simulink model "SecRwRtStLgrstUpwdDnwdTrgtPosSelc"  (R2018b)
settings: Solver=FixedStepDiscrete  StartTime=0.0  StopTime=10.0  FixedStep=0.01  RelTol=1e-3
undefined symbols (not defined in the file or in its folder): KeSMSw4SAcsMd24SecRwRtStLegrstUpwdDnwdPos_Val, KeSMSw4SAcsMd24SecRwRtStLegrstUpwdDnwdPosMax_Val, KeSMSw4SAcsMd24SecRwRtStLegrstUpwdDnwdPosMin_Val, KeSMSw4SAcsMd26SecRwRtStLegrstUpwdDnwdPos_Val, KeSMSw4SAcsMd26SecRwRtStLegrstUpwdDnwdPosMax_Val, KeSMSw4SAcsMd26SecRwRtStLegrstUpwdDnwdPosMin_Val, KeSMSw4SLegrstCloseMdSecRwRtStLgrstUpwdDnwdPos_Val, KeSMSw4SLegrstCloseMdSecRwRtStLgrstUpwdDnwdPosMax_Val, KeSMSw4SLegrstCloseMdSecRwRtStLgrstUpwdDnwdPosMin_Val, KeSMSw4SLegrstOpenMdSecRwRtStLgrstUpwdDnwdPos_Val, KeSMSw4SLegrstOpenMdSecRwRtStLgrstUpwdDnwdPosMax_Val, KeSMSw4SLegrstOpenMdSecRwRtStLgrstUpwdDnwdPosMin_Val, KeSMSw4sLyingMDSecRwRtStLgrstUpwdPos_Val, KeSMSw4sLyingMDSecRwRtStLgrstUpwdPosMax_Val, KeSMSw4sLyingMDSecRwRtStLgrstUpwdPosMin_Val, KeSMSw4sRecoveryMDSecRwRtStLgrstUpwdPos_Val, KeSMSw4sRecoveryMDSecRwRtStLgrstUpwdPosMax_Val, KeSMSw4sRecoveryMDSecRwRtStLgrstUpwdPosMin_Val, KeSMSw4sVIPMDSecRwRtStLgrstUpwdPos_Val, KeSMSw4sVIPMDSecRwRtStLgrstUpwdPosMax_Val, KeSMSw4sVIPMDSecRwRtStLgrstUpwdPosMin_Val, KeSMSw6sAcsEntrySecRwRtStLgrstUpwdPos_Val, KeSMSw6sAcsEntrySecRwRtStLgrstUpwdPosMax_Val, KeSMSw6sAcsEntrySecRwRtStLgrstUpwdPosMin_Val, KeSMSw6sAcsExtSecRwRtStLgrstUpwdDnwdPos_Val, KeSMSw6sAcsExtSecRwRtStLgrstUpwdDnwdPosMax_Val, KeSMSw6sAcsExtSecRwRtStLgrstUpwdDnwdPosMin_Val, KeSMSw6sRecoveryMdSecRwRtStLgrstUpwdDnwdPos_Val, KeSMSw6sRecoveryMdSecRwRtStLgrstUpwdDnwdPosMax_Val, KeSMSw6sRecoveryMdSecRwRtStLgrstUpwdDnwdPosMin_Val, KeSMSw6sVIPSecRwRtStLgrstUpwdPos_Val, KeSMSw6sVIPSecRwRtStLgrstUpwdPosMax_Val, KeSMSw6sVIPSecRwRtStLgrstUpwdPosMin_Val, KeSMSwAcsEntrySecRwRtStLgrstUpwdPos_Val, KeSMSwAcsEntrySecRwRtStLgrstUpwdPosMax_Val, KeSMSwAcsEntrySecRwRtStLgrstUpwdPosMin_Val, KeSMSwAcsExtSecRwRtStLgrstUpwdDnwdPos_Val, KeSMSwAcsExtSecRwRtStLgrstUpwdDnwdPosMax_Val, KeSMSwAcsExtSecRwRtStLgrstUpwdDnwdPosMin_Val, KeSMSwAcsMd8SecRwRtStLgrstUpwdPos_Val, KeSMSwAcsMd8SecRwRtStLgrstUpwdPosMax_Val, KeSMSwAcsMd8SecRwRtStLgrstUpwdPosMin_Val, KeSMSwAcsMd9SecRwRtStLgrstUpwdPos_Val, KeSMSwAcsMd9SecRwRtStLgrstUpwdPosMax_Val, KeSMSwAcsMd9SecRwRtStLgrstUpwdPosMin_Val, KeSMSwRecoveryMdSecRwRtStLgrstUpwdDnwdPos_Val, KeSMSwRecoveryMdSecRwRtStLgrstUpwdDnwdPosMax_Val, KeSMSwRecoveryMdSecRwRtStLgrstUpwdDnwdPosMin_Val, KeSMSwVIPSecRwRtStLgrstUpwdPos_Val, KeSMSwVIPSecRwRtStLgrstUpwdPosMax_Val, KeSMSwVIPSecRwRtStLgrstUpwdPosMin_Val
libraries: TrgtPosSelcLib x12
settings Model: Creator=sn2xws  LastModifiedBy=sn2xws
settings Model: ModifiedHistory=|
  | 2023.8.1 V2.0.0 CR421790 增加模式21-26
  | 2024.7.8 V3.0.0 557模式流程V1.9
settings DataIOCC: SaveFormat=StructureWithTime
settings OptimizationCC: DefaultParameterBehavior=Inlined  EnhancedBackFolding=on  PassReuseOutputArgsAs=Individual arguments  ZeroExternalMemoryAtStartup=off  ZeroInternalMemoryAtStartup=off  OptimizeBlockOrder=speed  DifferentSizesBufferReuse=on  OptimizationCustomize=off
settings DebuggingCC: ParameterTunabilityLossMsg=error
settings ModelReferenceCC: ModelReferenceNumInstancesAllowed=Single
settings SFSimCC: MATLABDynamicMemAlloc=off
settings RTWCC: SystemTargetFile=autosar.tlc  GenCodeOnly=on  TemplateMakefile=ert_default_tmf  Description=AUTOSAR  GenerateReport=on  IncludeHyperlinkInReport=on  LaunchReport=on  GenerateTraceInfo=on  GenerateTraceReport=on  GenerateTraceReportSl=on  GenerateTraceReportSf=on  GenerateTraceReportEml=on
settings CodeAppCC: ForceParamTrailComments=on  IgnoreCustomStorageClasses=off  OperatorAnnotations=on  SimulinkDataObjDesc=on  SFDataObjDesc=on  InsertBlockDesc=on
settings STFCustomTargetCC: TargetLangStandard=C99 (ISO)  MultiwordLength=256  ParMdlRefBuildCompliant=on  CompOptLevelCompliant=on  IncludeMdlTerminateFcn=off  CombineOutputUpdateFcns=on  SuppressErrorStatus=on  ERTCustomFileBanners=on  SupportNonFinite=off  SupportComplex=off  SupportContinuousTime=off  SupportNonInlinedSFcns=off  RemoveResetFunc=on  MATLABClassNameForMDSCustomization=Simulink.SoftwareTarget.ERTCustomization  AutosarCompliant=on  UseToolchainInfoCompliant=on  LookupTableObjectStructAxisOrder=2,1,3,4,...  LUTObjectStructOrderEvenSpacing=Size,Table,Breakpoints  SystemTargetFile=autosar.tlc
settings ERTTargetCC: TargetLangStandard=C99 (ISO)  ConcurrentExecutionCompliant=off  IncludeMdlTerminateFcn=off  SuppressErrorStatus=on  SupportNonFinite=off  SupportComplex=off  ModelStepFunctionPrototypeControlCompliant=off  CPPClassGenCompliant=off  AutosarCompliant=on  LookupTableObjectStructAxisOrder=2,1,3,4,...  LUTObjectStructOrderEvenSpacing=Size,Table,Breakpoints  InlinedParameterPlacement=NonHierarchical  ERTCustomFileTemplate=example_file_process.tlc  ERTFilePackagingFormat=Compact

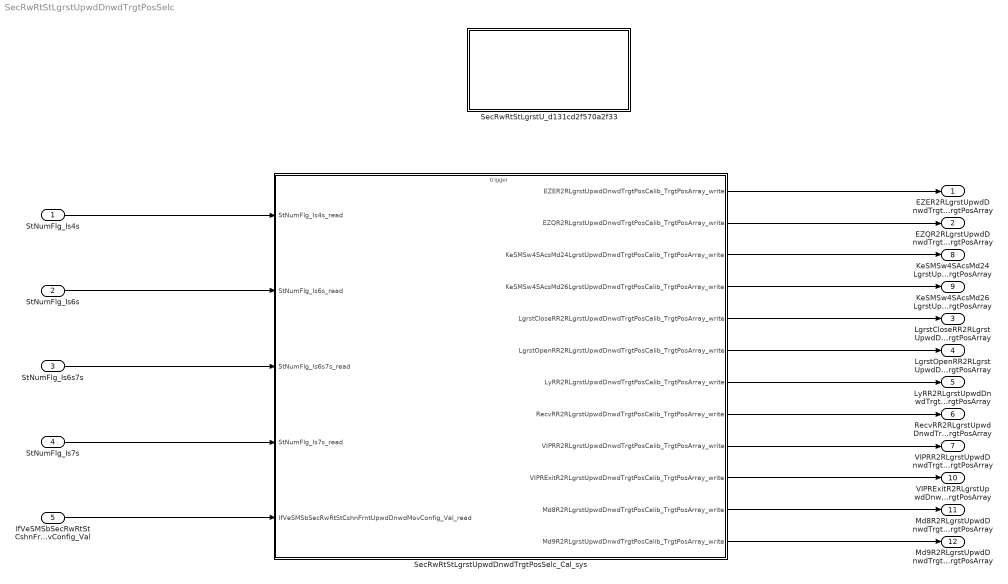
== system SecRwRtStLgrstUpwdDnwdTrgtPosSelc ==
  StNumFlg_Is4s : Inport  OutDataTypeStr=boolean  PortDimensions=1
  StNumFlg_Is6s : Inport  Port=2  OutDataTypeStr=boolean  PortDimensions=1
  StNumFlg_Is6s7s : Inport  Port=3  OutDataTypeStr=boolean  PortDimensions=1
  StNumFlg_Is7s : Inport  Port=4  OutDataTypeStr=boolean  PortDimensions=1
  IfVeSMSbSecRwRtStCshnFrntUpwdDnwdMovConfig_Val : Inport  Port=5  OutDataTypeStr=boolean  PortDimensions=1
  SecRwRtStLgrstU_d131cd2f570a2f33 : Subsystem
  SecRwRtStLgrstUpwdDnwdTrgtPosSelc_Cal_sys : Subsystem
  EZER2RLgrstUpwdDnwdTrgtPosCalib_TrgtPosArray : Outport  Description=|  OutDataTypeStr=uint16  PortDimensions=3
      | 0:Pos
      | 1:Max
      | 2:Min
  EZQR2RLgrstUpwdDnwdTrgtPosCalib_TrgtPosArray : Outport  Description=|  Port=2  OutDataTypeStr=uint16  PortDimensions=3
      | 0:Pos
      | 1:Max
      | 2:Min
  LgrstCloseRR2RLgrstUpwdDnwdTrgtPosCalib_TrgtPosArray : Outport  Description=|  Port=3  OutDataTypeStr=uint16  PortDimensions=3
      | 0:Pos
      | 1:Max
      | 2:Min
  LgrstOpenRR2RLgrstUpwdDnwdTrgtPosCalib_TrgtPosArray : Outport  Description=|  Port=4  OutDataTypeStr=uint16  PortDimensions=3
      | 0:Pos
      | 1:Max
      | 2:Min
  LyRR2RLgrstUpwdDnwdTrgtPosCalib_TrgtPosArray : Outport  Description=|  Port=5  OutDataTypeStr=uint16  PortDimensions=3
      | 0:Pos
      | 1:Max
      | 2:Min
  RecvRR2RLgrstUpwdDnwdTrgtPosCalib_TrgtPosArray : Outport  Description=|  Port=6  OutDataTypeStr=uint16  PortDimensions=3
      | 0:Pos
      | 1:Max
      | 2:Min
  VIPRR2RLgrstUpwdDnwdTrgtPosCalib_TrgtPosArray : Outport  Description=|  Port=7  OutDataTypeStr=uint16  PortDimensions=3
      | 0:Pos
      | 1:Max
      | 2:Min
  KeSMSw4SAcsMd24LgrstUpwdDnwdTrgtPosCalib_TrgtPosArray : Outport  Description=|  Port=8  OutDataTypeStr=uint16  PortDimensions=3
      | 0:Pos
      | 1:Max
      | 2:Min
  KeSMSw4SAcsMd26LgrstUpwdDnwdTrgtPosCalib_TrgtPosArray : Outport  Description=|  Port=9  OutDataTypeStr=uint16  PortDimensions=3
      | 0:Pos
      | 1:Max
      | 2:Min
  VIPRExitR2RLgrstUpwdDnwdTrgtPosCalib_TrgtPosArray : Outport  Description=|  Port=10  OutDataTypeStr=uint16  PortDimensions=3
      | 0:Pos
      | 1:Max
      | 2:Min
  Md8R2RLgrstUpwdDnwdTrgtPosCalib_TrgtPosArray : Outport  Description=|  Port=11  OutDataTypeStr=uint16  PortDimensions=3
      | 0:Pos
      | 1:Max
      | 2:Min
  Md9R2RLgrstUpwdDnwdTrgtPosCalib_TrgtPosArray : Outport  Description=|  Port=12  OutDataTypeStr=uint16  PortDimensions=3
      | 0:Pos
      | 1:Max
      | 2:Min
  wires:
  StNumFlg_Is4s/1 -> SecRwRtStLgrstUpwdDnwdTrgtPosSelc_Cal_sys/1(StNumFlg_Is4s_read)
  StNumFlg_Is6s/1 -> SecRwRtStLgrstUpwdDnwdTrgtPosSelc_Cal_sys/2(StNumFlg_Is6s_read)
  StNumFlg_Is6s7s/1 -> SecRwRtStLgrstUpwdDnwdTrgtPosSelc_Cal_sys/3(StNumFlg_Is6s7s_read)
  StNumFlg_Is7s/1 -> SecRwRtStLgrstUpwdDnwdTrgtPosSelc_Cal_sys/4(StNumFlg_Is7s_read)
  SecRwRtStLgrstUpwdDnwdTrgtPosSelc_Cal_sys/1(EZER2RLgrstUpwdDnwdTrgtPosCalib_TrgtPosArray_write) -> EZER2RLgrstUpwdDnwdTrgtPosCalib_TrgtPosArray/1
  SecRwRtStLgrstUpwdDnwdTrgtPosSelc_Cal_sys/2(EZQR2RLgrstUpwdDnwdTrgtPosCalib_TrgtPosArray_write) -> EZQR2RLgrstUpwdDnwdTrgtPosCalib_TrgtPosArray/1
  SecRwRtStLgrstUpwdDnwdTrgtPosSelc_Cal_sys/5(LgrstCloseRR2RLgrstUpwdDnwdTrgtPosCalib_TrgtPosArray_write) -> LgrstCloseRR2RLgrstUpwdDnwdTrgtPosCalib_TrgtPosArray/1
  SecRwRtStLgrstUpwdDnwdTrgtPosSelc_Cal_sys/6(LgrstOpenRR2RLgrstUpwdDnwdTrgtPosCalib_TrgtPosArray_write) -> LgrstOpenRR2RLgrstUpwdDnwdTrgtPosCalib_TrgtPosArray/1
  SecRwRtStLgrstUpwdDnwdTrgtPosSelc_Cal_sys/7(LyRR2RLgrstUpwdDnwdTrgtPosCalib_TrgtPosArray_write) -> LyRR2RLgrstUpwdDnwdTrgtPosCalib_TrgtPosArray/1
  SecRwRtStLgrstUpwdDnwdTrgtPosSelc_Cal_sys/8(RecvRR2RLgrstUpwdDnwdTrgtPosCalib_TrgtPosArray_write) -> RecvRR2RLgrstUpwdDnwdTrgtPosCalib_TrgtPosArray/1
  SecRwRtStLgrstUpwdDnwdTrgtPosSelc_Cal_sys/9(VIPRR2RLgrstUpwdDnwdTrgtPosCalib_TrgtPosArray_write) -> VIPRR2RLgrstUpwdDnwdTrgtPosCalib_TrgtPosArray/1
  SecRwRtStLgrstUpwdDnwdTrgtPosSelc_Cal_sys/3(KeSMSw4SAcsMd24LgrstUpwdDnwdTrgtPosCalib_TrgtPosArray_write) -> KeSMSw4SAcsMd24LgrstUpwdDnwdTrgtPosCalib_TrgtPosArray/1
  SecRwRtStLgrstUpwdDnwdTrgtPosSelc_Cal_sys/4(KeSMSw4SAcsMd26LgrstUpwdDnwdTrgtPosCalib_TrgtPosArray_write) -> KeSMSw4SAcsMd26LgrstUpwdDnwdTrgtPosCalib_TrgtPosArray/1
  IfVeSMSbSecRwRtStCshnFrntUpwdDnwdMovConfig_Val/1 -> SecRwRtStLgrstUpwdDnwdTrgtPosSelc_Cal_sys/5(IfVeSMSbSecRwRtStCshnFrntUpwdDnwdMovConfig_Val_read)
  SecRwRtStLgrstUpwdDnwdTrgtPosSelc_Cal_sys/10(VIPRExitR2RLgrstUpwdDnwdTrgtPosCalib_TrgtPosArray_write) -> VIPRExitR2RLgrstUpwdDnwdTrgtPosCalib_TrgtPosArray/1
  SecRwRtStLgrstUpwdDnwdTrgtPosSelc_Cal_sys/11(Md8R2RLgrstUpwdDnwdTrgtPosCalib_TrgtPosArray_write) -> Md8R2RLgrstUpwdDnwdTrgtPosCalib_TrgtPosArray/1
  SecRwRtStLgrstUpwdDnwdTrgtPosSelc_Cal_sys/12(Md9R2RLgrstUpwdDnwdTrgtPosCalib_TrgtPosArray_write) -> Md9R2RLgrstUpwdDnwdTrgtPosCalib_TrgtPosArray/1

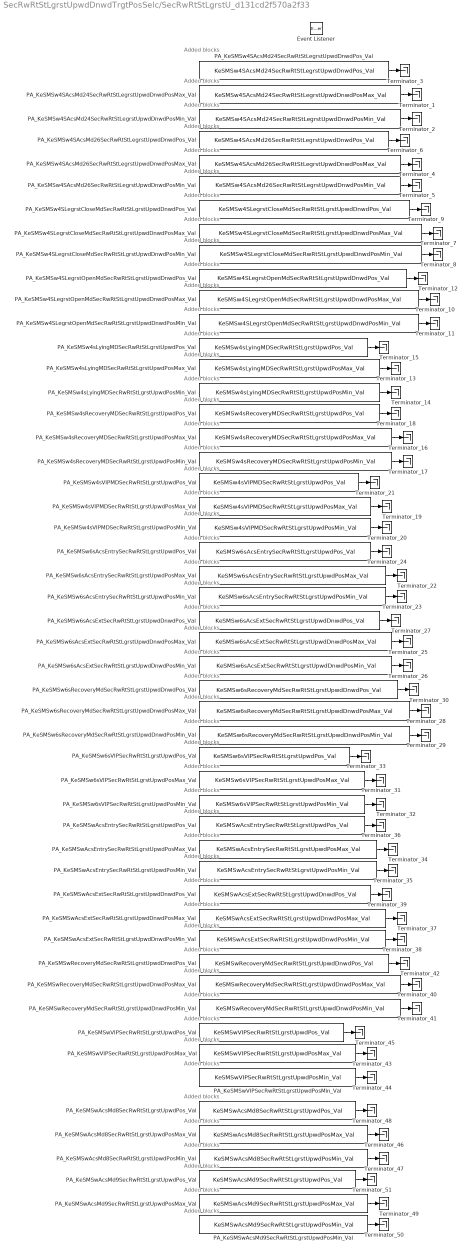
== system SecRwRtStLgrstUpwdDnwdTrgtPosSelc/SecRwRtStLgrstU_d131cd2f570a2f33 ==
  note: Added blocks
  note: Added blocks
  note: Added blocks
  note: Added blocks
  note: Added blocks
  note: Added blocks
  note: Added blocks
  note: Added blocks
  note: Added blocks
  note: Added blocks
  note: Added blocks
  note: Added blocks
  note: Added blocks
  note: Added blocks
  note: Added blocks
  note: Added blocks
  note: Added blocks
  note: Added blocks
  note: Added blocks
  note: Added blocks
  note: Added blocks
  note: Added blocks
  note: Added blocks
  note: Added blocks
  note: Added blocks
  note: Added blocks
  note: Added blocks
  note: Added blocks
  note: Added blocks
  note: Added blocks
  note: Added blocks
  note: Added blocks
  note: Added blocks
  note: Added blocks
  note: Added blocks
  note: Added blocks
  note: Added blocks
  note: Added blocks
  note: Added blocks
  note: Added blocks
  note: Added blocks
  note: Added blocks
  note: Added blocks
  note: Added blocks
  note: Added blocks
  note: Added blocks
  note: Added blocks
  note: Added blocks
  note: Added blocks
  note: Added blocks
  note: Added blocks
  Event Listener : EventListener  EventName=reset
  PA_KeSMSw4SAcsMd24SecRwRtStLegrstUpwdDnwdPosMax_Val : Constant  Value=KeSMSw4SAcsMd24SecRwRtStLegrstUpwdDnwdPosMax_Val
  PA_KeSMSw4SAcsMd24SecRwRtStLegrstUpwdDnwdPosMin_Val : Constant  Value=KeSMSw4SAcsMd24SecRwRtStLegrstUpwdDnwdPosMin_Val
  PA_KeSMSw4SAcsMd24SecRwRtStLegrstUpwdDnwdPos_Val : Constant  Value=KeSMSw4SAcsMd24SecRwRtStLegrstUpwdDnwdPos_Val
  PA_KeSMSw4SAcsMd26SecRwRtStLegrstUpwdDnwdPosMax_Val : Constant  Value=KeSMSw4SAcsMd26SecRwRtStLegrstUpwdDnwdPosMax_Val
  PA_KeSMSw4SAcsMd26SecRwRtStLegrstUpwdDnwdPosMin_Val : Constant  Value=KeSMSw4SAcsMd26SecRwRtStLegrstUpwdDnwdPosMin_Val
  PA_KeSMSw4SAcsMd26SecRwRtStLegrstUpwdDnwdPos_Val : Constant  Value=KeSMSw4SAcsMd26SecRwRtStLegrstUpwdDnwdPos_Val
  PA_KeSMSw4SLegrstCloseMdSecRwRtStLgrstUpwdDnwdPosMax_Val : Constant  Value=KeSMSw4SLegrstCloseMdSecRwRtStLgrstUpwdDnwdPosMax_Val
  PA_KeSMSw4SLegrstCloseMdSecRwRtStLgrstUpwdDnwdPosMin_Val : Constant  Value=KeSMSw4SLegrstCloseMdSecRwRtStLgrstUpwdDnwdPosMin_Val
  PA_KeSMSw4SLegrstCloseMdSecRwRtStLgrstUpwdDnwdPos_Val : Constant  Value=KeSMSw4SLegrstCloseMdSecRwRtStLgrstUpwdDnwdPos_Val
  PA_KeSMSw4SLegrstOpenMdSecRwRtStLgrstUpwdDnwdPosMax_Val : Constant  Value=KeSMSw4SLegrstOpenMdSecRwRtStLgrstUpwdDnwdPosMax_Val
  PA_KeSMSw4SLegrstOpenMdSecRwRtStLgrstUpwdDnwdPosMin_Val : Constant  Value=KeSMSw4SLegrstOpenMdSecRwRtStLgrstUpwdDnwdPosMin_Val
  PA_KeSMSw4SLegrstOpenMdSecRwRtStLgrstUpwdDnwdPos_Val : Constant  Value=KeSMSw4SLegrstOpenMdSecRwRtStLgrstUpwdDnwdPos_Val
  PA_KeSMSw4sLyingMDSecRwRtStLgrstUpwdPosMax_Val : Constant  Value=KeSMSw4sLyingMDSecRwRtStLgrstUpwdPosMax_Val
  PA_KeSMSw4sLyingMDSecRwRtStLgrstUpwdPosMin_Val : Constant  Value=KeSMSw4sLyingMDSecRwRtStLgrstUpwdPosMin_Val
  PA_KeSMSw4sLyingMDSecRwRtStLgrstUpwdPos_Val : Constant  Value=KeSMSw4sLyingMDSecRwRtStLgrstUpwdPos_Val
  PA_KeSMSw4sRecoveryMDSecRwRtStLgrstUpwdPosMax_Val : Constant  Value=KeSMSw4sRecoveryMDSecRwRtStLgrstUpwdPosMax_Val
  PA_KeSMSw4sRecoveryMDSecRwRtStLgrstUpwdPosMin_Val : Constant  Value=KeSMSw4sRecoveryMDSecRwRtStLgrstUpwdPosMin_Val
  PA_KeSMSw4sRecoveryMDSecRwRtStLgrstUpwdPos_Val : Constant  Value=KeSMSw4sRecoveryMDSecRwRtStLgrstUpwdPos_Val
  PA_KeSMSw4sVIPMDSecRwRtStLgrstUpwdPosMax_Val : Constant  Value=KeSMSw4sVIPMDSecRwRtStLgrstUpwdPosMax_Val
  PA_KeSMSw4sVIPMDSecRwRtStLgrstUpwdPosMin_Val : Constant  Value=KeSMSw4sVIPMDSecRwRtStLgrstUpwdPosMin_Val
  PA_KeSMSw4sVIPMDSecRwRtStLgrstUpwdPos_Val : Constant  Value=KeSMSw4sVIPMDSecRwRtStLgrstUpwdPos_Val
  PA_KeSMSw6sAcsEntrySecRwRtStLgrstUpwdPosMax_Val : Constant  Value=KeSMSw6sAcsEntrySecRwRtStLgrstUpwdPosMax_Val
  PA_KeSMSw6sAcsEntrySecRwRtStLgrstUpwdPosMin_Val : Constant  Value=KeSMSw6sAcsEntrySecRwRtStLgrstUpwdPosMin_Val
  PA_KeSMSw6sAcsEntrySecRwRtStLgrstUpwdPos_Val : Constant  Value=KeSMSw6sAcsEntrySecRwRtStLgrstUpwdPos_Val
  PA_KeSMSw6sAcsExtSecRwRtStLgrstUpwdDnwdPosMax_Val : Constant  Value=KeSMSw6sAcsExtSecRwRtStLgrstUpwdDnwdPosMax_Val
  PA_KeSMSw6sAcsExtSecRwRtStLgrstUpwdDnwdPosMin_Val : Constant  Value=KeSMSw6sAcsExtSecRwRtStLgrstUpwdDnwdPosMin_Val
  PA_KeSMSw6sAcsExtSecRwRtStLgrstUpwdDnwdPos_Val : Constant  Value=KeSMSw6sAcsExtSecRwRtStLgrstUpwdDnwdPos_Val
  PA_KeSMSw6sRecoveryMdSecRwRtStLgrstUpwdDnwdPosMax_Val : Constant  Value=KeSMSw6sRecoveryMdSecRwRtStLgrstUpwdDnwdPosMax_Val
  PA_KeSMSw6sRecoveryMdSecRwRtStLgrstUpwdDnwdPosMin_Val : Constant  Value=KeSMSw6sRecoveryMdSecRwRtStLgrstUpwdDnwdPosMin_Val
  PA_KeSMSw6sRecoveryMdSecRwRtStLgrstUpwdDnwdPos_Val : Constant  Value=KeSMSw6sRecoveryMdSecRwRtStLgrstUpwdDnwdPos_Val
  PA_KeSMSw6sVIPSecRwRtStLgrstUpwdPosMax_Val : Constant  Value=KeSMSw6sVIPSecRwRtStLgrstUpwdPosMax_Val
  PA_KeSMSw6sVIPSecRwRtStLgrstUpwdPosMin_Val : Constant  Value=KeSMSw6sVIPSecRwRtStLgrstUpwdPosMin_Val
  PA_KeSMSw6sVIPSecRwRtStLgrstUpwdPos_Val : Constant  Value=KeSMSw6sVIPSecRwRtStLgrstUpwdPos_Val
  PA_KeSMSwAcsEntrySecRwRtStLgrstUpwdPosMax_Val : Constant  Value=KeSMSwAcsEntrySecRwRtStLgrstUpwdPosMax_Val
  PA_KeSMSwAcsEntrySecRwRtStLgrstUpwdPosMin_Val : Constant  Value=KeSMSwAcsEntrySecRwRtStLgrstUpwdPosMin_Val
  PA_KeSMSwAcsEntrySecRwRtStLgrstUpwdPos_Val : Constant  Value=KeSMSwAcsEntrySecRwRtStLgrstUpwdPos_Val
  PA_KeSMSwAcsExtSecRwRtStLgrstUpwdDnwdPosMax_Val : Constant  Value=KeSMSwAcsExtSecRwRtStLgrstUpwdDnwdPosMax_Val
  PA_KeSMSwAcsExtSecRwRtStLgrstUpwdDnwdPosMin_Val : Constant  Value=KeSMSwAcsExtSecRwRtStLgrstUpwdDnwdPosMin_Val
  PA_KeSMSwAcsExtSecRwRtStLgrstUpwdDnwdPos_Val : Constant  Value=KeSMSwAcsExtSecRwRtStLgrstUpwdDnwdPos_Val
  PA_KeSMSwAcsMd8SecRwRtStLgrstUpwdPosMax_Val : Constant  Value=KeSMSwAcsMd8SecRwRtStLgrstUpwdPosMax_Val
  PA_KeSMSwAcsMd8SecRwRtStLgrstUpwdPosMin_Val : Constant  Value=KeSMSwAcsMd8SecRwRtStLgrstUpwdPosMin_Val
  PA_KeSMSwAcsMd8SecRwRtStLgrstUpwdPos_Val : Constant  Value=KeSMSwAcsMd8SecRwRtStLgrstUpwdPos_Val
  PA_KeSMSwAcsMd9SecRwRtStLgrstUpwdPosMax_Val : Constant  Value=KeSMSwAcsMd9SecRwRtStLgrstUpwdPosMax_Val
  PA_KeSMSwAcsMd9SecRwRtStLgrstUpwdPosMin_Val : Constant  Value=KeSMSwAcsMd9SecRwRtStLgrstUpwdPosMin_Val
  PA_KeSMSwAcsMd9SecRwRtStLgrstUpwdPos_Val : Constant  Value=KeSMSwAcsMd9SecRwRtStLgrstUpwdPos_Val
  PA_KeSMSwRecoveryMdSecRwRtStLgrstUpwdDnwdPosMax_Val : Constant  Value=KeSMSwRecoveryMdSecRwRtStLgrstUpwdDnwdPosMax_Val
  PA_KeSMSwRecoveryMdSecRwRtStLgrstUpwdDnwdPosMin_Val : Constant  Value=KeSMSwRecoveryMdSecRwRtStLgrstUpwdDnwdPosMin_Val
  PA_KeSMSwRecoveryMdSecRwRtStLgrstUpwdDnwdPos_Val : Constant  Value=KeSMSwRecoveryMdSecRwRtStLgrstUpwdDnwdPos_Val
  PA_KeSMSwVIPSecRwRtStLgrstUpwdPosMax_Val : Constant  Value=KeSMSwVIPSecRwRtStLgrstUpwdPosMax_Val
  PA_KeSMSwVIPSecRwRtStLgrstUpwdPosMin_Val : Constant  Value=KeSMSwVIPSecRwRtStLgrstUpwdPosMin_Val
  PA_KeSMSwVIPSecRwRtStLgrstUpwdPos_Val : Constant  Value=KeSMSwVIPSecRwRtStLgrstUpwdPos_Val
  Terminator_{1..51} (51 alike) : Terminator
  wires:
  PA_KeSMSw4SAcsMd24SecRwRtStLegrstUpwdDnwdPosMax_Val/1 -> Terminator_1/1
  PA_KeSMSw4SAcsMd24SecRwRtStLegrstUpwdDnwdPosMin_Val/1 -> Terminator_2/1
  PA_KeSMSw4SAcsMd24SecRwRtStLegrstUpwdDnwdPos_Val/1 -> Terminator_3/1
  PA_KeSMSw4SAcsMd26SecRwRtStLegrstUpwdDnwdPosMax_Val/1 -> Terminator_4/1
  PA_KeSMSw4SAcsMd26SecRwRtStLegrstUpwdDnwdPosMin_Val/1 -> Terminator_5/1
  PA_KeSMSw4SAcsMd26SecRwRtStLegrstUpwdDnwdPos_Val/1 -> Terminator_6/1
  PA_KeSMSw4SLegrstCloseMdSecRwRtStLgrstUpwdDnwdPosMax_Val/1 -> Terminator_7/1
  PA_KeSMSw4SLegrstCloseMdSecRwRtStLgrstUpwdDnwdPosMin_Val/1 -> Terminator_8/1
  PA_KeSMSw4SLegrstCloseMdSecRwRtStLgrstUpwdDnwdPos_Val/1 -> Terminator_9/1
  PA_KeSMSw4SLegrstOpenMdSecRwRtStLgrstUpwdDnwdPosMax_Val/1 -> Terminator_10/1
  PA_KeSMSw4SLegrstOpenMdSecRwRtStLgrstUpwdDnwdPosMin_Val/1 -> Terminator_11/1
  PA_KeSMSw4SLegrstOpenMdSecRwRtStLgrstUpwdDnwdPos_Val/1 -> Terminator_12/1
  PA_KeSMSw4sLyingMDSecRwRtStLgrstUpwdPosMax_Val/1 -> Terminator_13/1
  PA_KeSMSw4sLyingMDSecRwRtStLgrstUpwdPosMin_Val/1 -> Terminator_14/1
  PA_KeSMSw4sLyingMDSecRwRtStLgrstUpwdPos_Val/1 -> Terminator_15/1
  PA_KeSMSw4sRecoveryMDSecRwRtStLgrstUpwdPosMax_Val/1 -> Terminator_16/1
  PA_KeSMSw4sRecoveryMDSecRwRtStLgrstUpwdPosMin_Val/1 -> Terminator_17/1
  PA_KeSMSw4sRecoveryMDSecRwRtStLgrstUpwdPos_Val/1 -> Terminator_18/1
  PA_KeSMSw4sVIPMDSecRwRtStLgrstUpwdPosMax_Val/1 -> Terminator_19/1
  PA_KeSMSw4sVIPMDSecRwRtStLgrstUpwdPosMin_Val/1 -> Terminator_20/1
  PA_KeSMSw4sVIPMDSecRwRtStLgrstUpwdPos_Val/1 -> Terminator_21/1
  PA_KeSMSw6sAcsEntrySecRwRtStLgrstUpwdPosMax_Val/1 -> Terminator_22/1
  PA_KeSMSw6sAcsEntrySecRwRtStLgrstUpwdPosMin_Val/1 -> Terminator_23/1
  PA_KeSMSw6sAcsEntrySecRwRtStLgrstUpwdPos_Val/1 -> Terminator_24/1
  PA_KeSMSw6sAcsExtSecRwRtStLgrstUpwdDnwdPosMax_Val/1 -> Terminator_25/1
  PA_KeSMSw6sAcsExtSecRwRtStLgrstUpwdDnwdPosMin_Val/1 -> Terminator_26/1
  PA_KeSMSw6sAcsExtSecRwRtStLgrstUpwdDnwdPos_Val/1 -> Terminator_27/1
  PA_KeSMSw6sRecoveryMdSecRwRtStLgrstUpwdDnwdPosMax_Val/1 -> Terminator_28/1
  PA_KeSMSw6sRecoveryMdSecRwRtStLgrstUpwdDnwdPosMin_Val/1 -> Terminator_29/1
  PA_KeSMSw6sRecoveryMdSecRwRtStLgrstUpwdDnwdPos_Val/1 -> Terminator_30/1
  PA_KeSMSw6sVIPSecRwRtStLgrstUpwdPosMax_Val/1 -> Terminator_31/1
  PA_KeSMSw6sVIPSecRwRtStLgrstUpwdPosMin_Val/1 -> Terminator_32/1
  PA_KeSMSw6sVIPSecRwRtStLgrstUpwdPos_Val/1 -> Terminator_33/1
  PA_KeSMSwAcsEntrySecRwRtStLgrstUpwdPosMax_Val/1 -> Terminator_34/1
  PA_KeSMSwAcsEntrySecRwRtStLgrstUpwdPosMin_Val/1 -> Terminator_35/1
  PA_KeSMSwAcsEntrySecRwRtStLgrstUpwdPos_Val/1 -> Terminator_36/1
  PA_KeSMSwAcsExtSecRwRtStLgrstUpwdDnwdPosMax_Val/1 -> Terminator_37/1
  PA_KeSMSwAcsExtSecRwRtStLgrstUpwdDnwdPosMin_Val/1 -> Terminator_38/1
  PA_KeSMSwAcsExtSecRwRtStLgrstUpwdDnwdPos_Val/1 -> Terminator_39/1
  PA_KeSMSwRecoveryMdSecRwRtStLgrstUpwdDnwdPosMax_Val/1 -> Terminator_40/1
  PA_KeSMSwRecoveryMdSecRwRtStLgrstUpwdDnwdPosMin_Val/1 -> Terminator_41/1
  PA_KeSMSwRecoveryMdSecRwRtStLgrstUpwdDnwdPos_Val/1 -> Terminator_42/1
  PA_KeSMSwVIPSecRwRtStLgrstUpwdPosMax_Val/1 -> Terminator_43/1
  PA_KeSMSwVIPSecRwRtStLgrstUpwdPosMin_Val/1 -> Terminator_44/1
  PA_KeSMSwVIPSecRwRtStLgrstUpwdPos_Val/1 -> Terminator_45/1
  PA_KeSMSwAcsMd8SecRwRtStLgrstUpwdPosMax_Val/1 -> Terminator_46/1
  PA_KeSMSwAcsMd8SecRwRtStLgrstUpwdPosMin_Val/1 -> Terminator_47/1
  PA_KeSMSwAcsMd8SecRwRtStLgrstUpwdPos_Val/1 -> Terminator_48/1
  PA_KeSMSwAcsMd9SecRwRtStLgrstUpwdPosMax_Val/1 -> Terminator_49/1
  PA_KeSMSwAcsMd9SecRwRtStLgrstUpwdPosMin_Val/1 -> Terminator_50/1
  PA_KeSMSwAcsMd9SecRwRtStLgrstUpwdPos_Val/1 -> Terminator_51/1

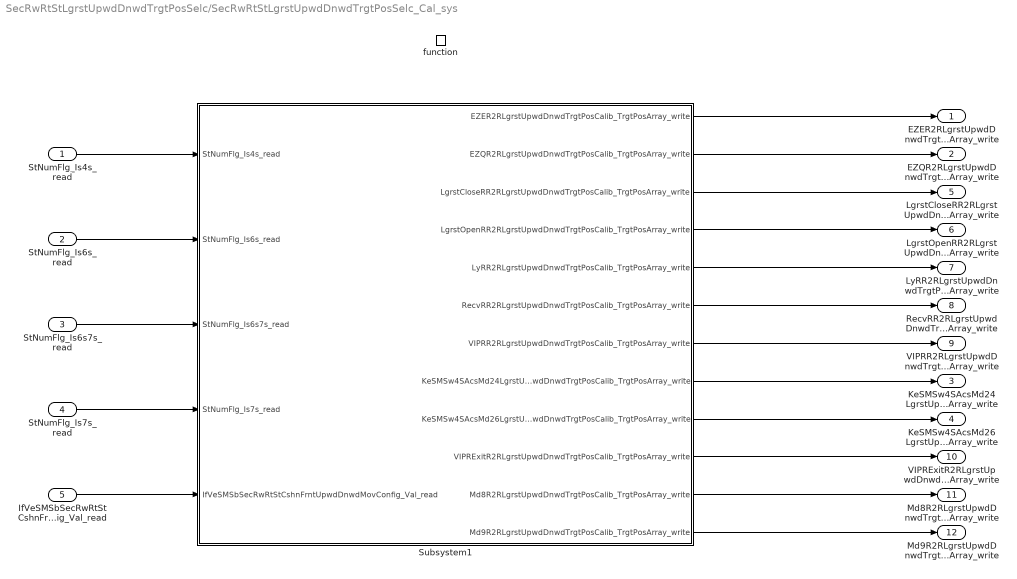
== system SecRwRtStLgrstUpwdDnwdTrgtPosSelc/SecRwRtStLgrstUpwdDnwdTrgtPosSelc_Cal_sys ==
  StNumFlg_Is4s_read : Inport
  StNumFlg_Is6s_read : Inport  Port=2
  StNumFlg_Is6s7s_read : Inport  Port=3
  StNumFlg_Is7s_read : Inport  Port=4
  IfVeSMSbSecRwRtStCshnFrntUpwdDnwdMovConfig_Val_read : Inport  Port=5
  function : TriggerPort  TriggerType=function-call  IsSimulinkFunction=on  FunctionName=SecRwRtStLgrstUpwdDnwdTrgtPosSelc_Cal  VariantControl=(inherit)
  Subsystem1 : Subsystem
  EZER2RLgrstUpwdDnwdTrgtPosCalib_TrgtPosArray_write : Outport
      settings: EnsureOutportIsVirtual=on
  EZQR2RLgrstUpwdDnwdTrgtPosCalib_TrgtPosArray_write : Outport  Port=2
      settings: EnsureOutportIsVirtual=on
  KeSMSw4SAcsMd24LgrstUpwdDnwdTrgtPosCalib_TrgtPosArray_write : Outport  Port=3
      settings: EnsureOutportIsVirtual=on
  KeSMSw4SAcsMd26LgrstUpwdDnwdTrgtPosCalib_TrgtPosArray_write : Outport  Port=4
      settings: EnsureOutportIsVirtual=on
  LgrstCloseRR2RLgrstUpwdDnwdTrgtPosCalib_TrgtPosArray_write : Outport  Port=5
      settings: EnsureOutportIsVirtual=on
  LgrstOpenRR2RLgrstUpwdDnwdTrgtPosCalib_TrgtPosArray_write : Outport  Port=6
      settings: EnsureOutportIsVirtual=on
  LyRR2RLgrstUpwdDnwdTrgtPosCalib_TrgtPosArray_write : Outport  Port=7
      settings: EnsureOutportIsVirtual=on
  RecvRR2RLgrstUpwdDnwdTrgtPosCalib_TrgtPosArray_write : Outport  Port=8
      settings: EnsureOutportIsVirtual=on
  VIPRR2RLgrstUpwdDnwdTrgtPosCalib_TrgtPosArray_write : Outport  Port=9
      settings: EnsureOutportIsVirtual=on
  VIPRExitR2RLgrstUpwdDnwdTrgtPosCalib_TrgtPosArray_write : Outport  Port=10
      settings: EnsureOutportIsVirtual=on
  Md8R2RLgrstUpwdDnwdTrgtPosCalib_TrgtPosArray_write : Outport  Port=11
      settings: EnsureOutportIsVirtual=on
  Md9R2RLgrstUpwdDnwdTrgtPosCalib_TrgtPosArray_write : Outport  Port=12
      settings: EnsureOutportIsVirtual=on
  wires:
  Subsystem1/1(EZER2RLgrstUpwdDnwdTrgtPosCalib_TrgtPosArray_write) -> EZER2RLgrstUpwdDnwdTrgtPosCalib_TrgtPosArray_write/1
  Subsystem1/2(EZQR2RLgrstUpwdDnwdTrgtPosCalib_TrgtPosArray_write) -> EZQR2RLgrstUpwdDnwdTrgtPosCalib_TrgtPosArray_write/1
  Subsystem1/7(VIPRR2RLgrstUpwdDnwdTrgtPosCalib_TrgtPosArray_write) -> VIPRR2RLgrstUpwdDnwdTrgtPosCalib_TrgtPosArray_write/1
  Subsystem1/8(KeSMSw4SAcsMd24LgrstUpwdDnwdTrgtPosCalib_TrgtPosArray_write) -> KeSMSw4SAcsMd24LgrstUpwdDnwdTrgtPosCalib_TrgtPosArray_write/1
  Subsystem1/4(LgrstOpenRR2RLgrstUpwdDnwdTrgtPosCalib_TrgtPosArray_write) -> LgrstOpenRR2RLgrstUpwdDnwdTrgtPosCalib_TrgtPosArray_write/1
  Subsystem1/5(LyRR2RLgrstUpwdDnwdTrgtPosCalib_TrgtPosArray_write) -> LyRR2RLgrstUpwdDnwdTrgtPosCalib_TrgtPosArray_write/1
  Subsystem1/6(RecvRR2RLgrstUpwdDnwdTrgtPosCalib_TrgtPosArray_write) -> RecvRR2RLgrstUpwdDnwdTrgtPosCalib_TrgtPosArray_write/1
  Subsystem1/9(KeSMSw4SAcsMd26LgrstUpwdDnwdTrgtPosCalib_TrgtPosArray_write) -> KeSMSw4SAcsMd26LgrstUpwdDnwdTrgtPosCalib_TrgtPosArray_write/1
  Subsystem1/3(LgrstCloseRR2RLgrstUpwdDnwdTrgtPosCalib_TrgtPosArray_write) -> LgrstCloseRR2RLgrstUpwdDnwdTrgtPosCalib_TrgtPosArray_write/1
  StNumFlg_Is4s_read/1 -> Subsystem1/1(StNumFlg_Is4s_read)
  StNumFlg_Is6s_read/1 -> Subsystem1/2(StNumFlg_Is6s_read)
  StNumFlg_Is6s7s_read/1 -> Subsystem1/3(StNumFlg_Is6s7s_read)
  StNumFlg_Is7s_read/1 -> Subsystem1/4(StNumFlg_Is7s_read)
  Subsystem1/10(VIPRExitR2RLgrstUpwdDnwdTrgtPosCalib_TrgtPosArray_write) -> VIPRExitR2RLgrstUpwdDnwdTrgtPosCalib_TrgtPosArray_write/1
  IfVeSMSbSecRwRtStCshnFrntUpwdDnwdMovConfig_Val_read/1 -> Subsystem1/5(IfVeSMSbSecRwRtStCshnFrntUpwdDnwdMovConfig_Val_read)
  Subsystem1/11(Md8R2RLgrstUpwdDnwdTrgtPosCalib_TrgtPosArray_write) -> Md8R2RLgrstUpwdDnwdTrgtPosCalib_TrgtPosArray_write/1
  Subsystem1/12(Md9R2RLgrstUpwdDnwdTrgtPosCalib_TrgtPosArray_write) -> Md9R2RLgrstUpwdDnwdTrgtPosCalib_TrgtPosArray_write/1

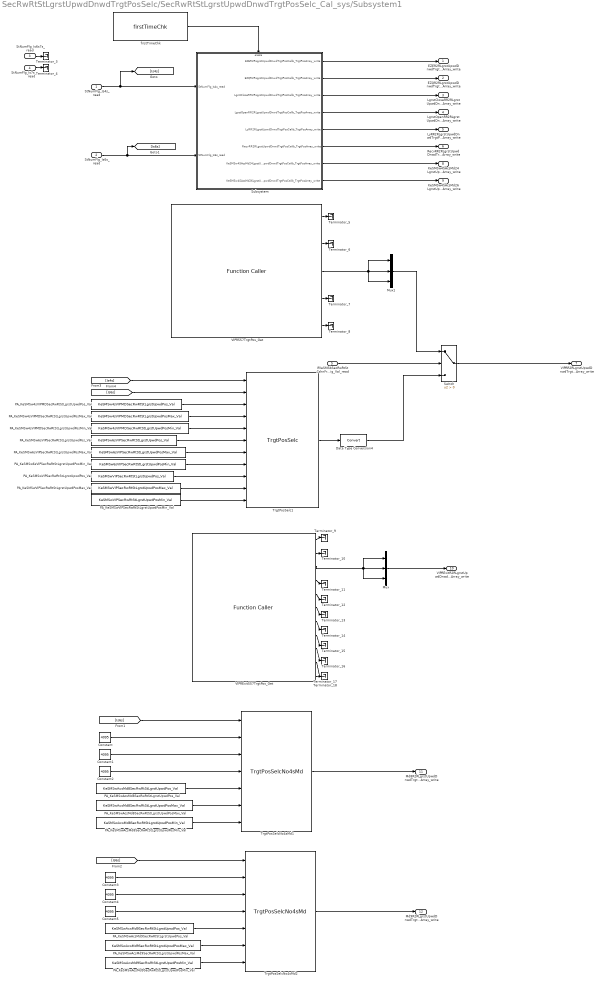
== system SecRwRtStLgrstUpwdDnwdTrgtPosSelc/SecRwRtStLgrstUpwdDnwdTrgtPosSelc_Cal_sys/Subsystem1 ==
  StNumFlg_Is4s_read : Inport
  StNumFlg_Is6s_read : Inport  Port=2
  StNumFlg_Is6s7s_read : Inport  Port=3
  StNumFlg_Is7s_read : Inport  Port=4
  IfVeSMSbSecRwRtStCshnFrntUpwdDnwdMovConfig_Val_read : Inport  Port=5
  Constant{,1..5} (6 alike) : Constant  Value=4095  OutDataTypeStr=uint16
  Data Type Conversion4 : DataTypeConversion
  Mux : Mux  Inputs=3
  Mux1 : Mux  Inputs=3
  PA_KeSMSw4sVIPMDSecRwRtStLgrstUpwdPosMax_Val : Constant  Value=KeSMSw4sVIPMDSecRwRtStLgrstUpwdPosMax_Val
  PA_KeSMSw4sVIPMDSecRwRtStLgrstUpwdPosMin_Val : Constant  Value=KeSMSw4sVIPMDSecRwRtStLgrstUpwdPosMin_Val
  PA_KeSMSw4sVIPMDSecRwRtStLgrstUpwdPos_Val : Constant  Value=KeSMSw4sVIPMDSecRwRtStLgrstUpwdPos_Val
  PA_KeSMSw6sVIPSecRwRtStLgrstUpwdPosMax_Val : Constant  Value=KeSMSw6sVIPSecRwRtStLgrstUpwdPosMax_Val
  PA_KeSMSw6sVIPSecRwRtStLgrstUpwdPosMin_Val : Constant  Value=KeSMSw6sVIPSecRwRtStLgrstUpwdPosMin_Val
  PA_KeSMSw6sVIPSecRwRtStLgrstUpwdPos_Val : Constant  Value=KeSMSw6sVIPSecRwRtStLgrstUpwdPos_Val
  PA_KeSMSwAcsMd8SecRwRtStLgrstUpwdPosMax_Val : Constant  Value=KeSMSwAcsMd8SecRwRtStLgrstUpwdPosMax_Val
  PA_KeSMSwAcsMd8SecRwRtStLgrstUpwdPosMin_Val : Constant  Value=KeSMSwAcsMd8SecRwRtStLgrstUpwdPosMin_Val
  PA_KeSMSwAcsMd8SecRwRtStLgrstUpwdPos_Val : Constant  Value=KeSMSwAcsMd8SecRwRtStLgrstUpwdPos_Val
  PA_KeSMSwAcsMd9SecRwRtStLgrstUpwdPosMax_Val : Constant  Value=KeSMSwAcsMd9SecRwRtStLgrstUpwdPosMax_Val
  PA_KeSMSwAcsMd9SecRwRtStLgrstUpwdPosMin_Val : Constant  Value=KeSMSwAcsMd9SecRwRtStLgrstUpwdPosMin_Val
  PA_KeSMSwAcsMd9SecRwRtStLgrstUpwdPos_Val : Constant  Value=KeSMSwAcsMd9SecRwRtStLgrstUpwdPos_Val
  PA_KeSMSwVIPSecRwRtStLgrstUpwdPosMax_Val : Constant  Value=KeSMSwVIPSecRwRtStLgrstUpwdPosMax_Val
  PA_KeSMSwVIPSecRwRtStLgrstUpwdPosMin_Val : Constant  Value=KeSMSwVIPSecRwRtStLgrstUpwdPosMin_Val
  PA_KeSMSwVIPSecRwRtStLgrstUpwdPos_Val : Constant  Value=KeSMSwVIPSecRwRtStLgrstUpwdPos_Val
  Subsystem : Subsystem
  Switch : Switch  Criteria=u2 > Threshold
  Terminator_{3..18} (16 alike) : Terminator
  TrgtPosSelc1 : TrgtPosSelcLib/TrgtPosSelc  SystemSampleTime=-1
  TrgtPosSelcNo4sMd1 : TrgtPosSelcLib/TrgtPosSelcNo4sMd  SystemSampleTime=-1
  TrgtPosSelcNo4sMd2 : TrgtPosSelcLib/TrgtPosSelcNo4sMd  SystemSampleTime=-1
  VIPR557TrgtPos_Get : FunctionCaller  FunctionPrototype=[SecRwLtStBkReclnTrgtPos,SecRwLtStZeroTrgtPos,SecRwLtStLgrstUpwdDnwdTrgtPos,SecRwLtStLgrstInwdOtwdTrgtPos,SecRwLtStFwdBkwdTrgtPos] = VIPR557TrgtPos_Get()  OutputArgumentSpecifications=uint16(1), uint16(1), uint16(1), uint16(1), uint16(1)
  VIPRExit557TrgtPos_Get : FunctionCaller  FunctionPrototype=[SecRwRtStBkReclnTrgtPos,SecRwRtStZeroTrgtPos,SecRwRtStLgrstUpwdDnwdTrgtPos,SecRwRtStLgrstInwdOtwdTrgtPos,ThdRwLtStBkReclnTrgtPos,ThdRwLtStFwdBkwdTrgtPos,ThdRwRtStBkReclnTrgtPos,ThdRwRtStFwdBkwdTrgtPos,PassStBkReclnTrgtPos,PassStFwdBkwdTrgtPos,SecRwRtStFwdBkwdTrgtPos] = VIPRExit557TrgtPos_Get()  OutputArgumentSpecifications=uint16(1), uint16(1), uint16(1), uint16(1), uint16(1), uint16(1), uint16(1), uint16(1), uint16(1), uint16(1), uint16(1)
  firstTimeChk : TrgtPosSelcLib/firstTimeChk  SystemSampleTime=-1
  EZER2RLgrstUpwdDnwdTrgtPosCalib_TrgtPosArray_write : Outport
      settings: EnsureOutportIsVirtual=on
  EZQR2RLgrstUpwdDnwdTrgtPosCalib_TrgtPosArray_write : Outport  Port=2
      settings: EnsureOutportIsVirtual=on
  LgrstCloseRR2RLgrstUpwdDnwdTrgtPosCalib_TrgtPosArray_write : Outport  Port=3
      settings: EnsureOutportIsVirtual=on
  LgrstOpenRR2RLgrstUpwdDnwdTrgtPosCalib_TrgtPosArray_write : Outport  Port=4
      settings: EnsureOutportIsVirtual=on
  LyRR2RLgrstUpwdDnwdTrgtPosCalib_TrgtPosArray_write : Outport  Port=5
      settings: EnsureOutportIsVirtual=on
  RecvRR2RLgrstUpwdDnwdTrgtPosCalib_TrgtPosArray_write : Outport  Port=6
      settings: EnsureOutportIsVirtual=on
  VIPRR2RLgrstUpwdDnwdTrgtPosCalib_TrgtPosArray_write : Outport  Port=7
      settings: EnsureOutportIsVirtual=on
  KeSMSw4SAcsMd24LgrstUpwdDnwdTrgtPosCalib_TrgtPosArray_write : Outport  Port=8
      settings: EnsureOutportIsVirtual=on
  KeSMSw4SAcsMd26LgrstUpwdDnwdTrgtPosCalib_TrgtPosArray_write : Outport  Port=9
      settings: EnsureOutportIsVirtual=on
  VIPRExitR2RLgrstUpwdDnwdTrgtPosCalib_TrgtPosArray_write : Outport  Port=10
      settings: EnsureOutportIsVirtual=on
  Md8R2RLgrstUpwdDnwdTrgtPosCalib_TrgtPosArray_write : Outport  Port=11
      settings: EnsureOutportIsVirtual=on
  Md9R2RLgrstUpwdDnwdTrgtPosCalib_TrgtPosArray_write : Outport  Port=12
      settings: EnsureOutportIsVirtual=on
  wires:
  StNumFlg_Is6s7s_read/1 -> Terminator_3/1
  Subsystem/2(EZQR2RLgrstUpwdDnwdTrgtPosCalib_TrgtPosArray_write) -> EZQR2RLgrstUpwdDnwdTrgtPosCalib_TrgtPosArray_write/1
  Subsystem/6(RecvRR2RLgrstUpwdDnwdTrgtPosCalib_TrgtPosArray_write) -> RecvRR2RLgrstUpwdDnwdTrgtPosCalib_TrgtPosArray_write/1
  Subsystem/3(LgrstCloseRR2RLgrstUpwdDnwdTrgtPosCalib_TrgtPosArray_write) -> LgrstCloseRR2RLgrstUpwdDnwdTrgtPosCalib_TrgtPosArray_write/1
  StNumFlg_Is7s_read/1 -> Terminator_4/1
  Subsystem/1(EZER2RLgrstUpwdDnwdTrgtPosCalib_TrgtPosArray_write) -> EZER2RLgrstUpwdDnwdTrgtPosCalib_TrgtPosArray_write/1
  Subsystem/5(LyRR2RLgrstUpwdDnwdTrgtPosCalib_TrgtPosArray_write) -> LyRR2RLgrstUpwdDnwdTrgtPosCalib_TrgtPosArray_write/1
  Subsystem/4(LgrstOpenRR2RLgrstUpwdDnwdTrgtPosCalib_TrgtPosArray_write) -> LgrstOpenRR2RLgrstUpwdDnwdTrgtPosCalib_TrgtPosArray_write/1
  firstTimeChk/1 -> Subsystem/Enable
  StNumFlg_Is6s_read/1 -> [Is6s], Subsystem/2(StNumFlg_Is6s_read)
  StNumFlg_Is4s_read/1 -> [Is4s], Subsystem/1(StNumFlg_Is4s_read)
  Subsystem/8(KeSMSw4SAcsMd26LgrstUpwdDnwdTrgtPosCalib_TrgtPosArray_write) -> KeSMSw4SAcsMd26LgrstUpwdDnwdTrgtPosCalib_TrgtPosArray_write/1
  Subsystem/7(KeSMSw4SAcsMd24LgrstUpwdDnwdTrgtPosCalib_TrgtPosArray_write) -> KeSMSw4SAcsMd24LgrstUpwdDnwdTrgtPosCalib_TrgtPosArray_write/1
  IfVeSMSbSecRwRtStCshnFrntUpwdDnwdMovConfig_Val_read/1 -> Switch/2
  Switch/1 -> VIPRR2RLgrstUpwdDnwdTrgtPosCalib_TrgtPosArray_write/1
  TrgtPosSelc1/1 -> Data Type Conversion4/1
  PA_KeSMSwVIPSecRwRtStLgrstUpwdPosMax_Val/1 -> TrgtPosSelc1/10
  PA_KeSMSw6sVIPSecRwRtStLgrstUpwdPosMin_Val/1 -> TrgtPosSelc1/8
  PA_KeSMSwVIPSecRwRtStLgrstUpwdPos_Val/1 -> TrgtPosSelc1/9
  PA_KeSMSw6sVIPSecRwRtStLgrstUpwdPosMax_Val/1 -> TrgtPosSelc1/7
  PA_KeSMSw6sVIPSecRwRtStLgrstUpwdPos_Val/1 -> TrgtPosSelc1/6
  [Is6s] -> TrgtPosSelc1/2
  PA_KeSMSw4sVIPMDSecRwRtStLgrstUpwdPosMax_Val/1 -> TrgtPosSelc1/4
  PA_KeSMSw4sVIPMDSecRwRtStLgrstUpwdPosMin_Val/1 -> TrgtPosSelc1/5
  PA_KeSMSw4sVIPMDSecRwRtStLgrstUpwdPos_Val/1 -> TrgtPosSelc1/3
  [Is4s] -> TrgtPosSelc1/1
  PA_KeSMSwVIPSecRwRtStLgrstUpwdPosMin_Val/1 -> TrgtPosSelc1/11
  Data Type Conversion4/1 -> Switch/3
  Mux/1 -> VIPRExitR2RLgrstUpwdDnwdTrgtPosCalib_TrgtPosArray_write/1
  VIPRExit557TrgtPos_Get/3 -> Mux/3, Mux/1, Mux/2
  Mux1/1 -> Switch/1
  VIPR557TrgtPos_Get/3 -> Mux1/3, Mux1/1, Mux1/2
  VIPR557TrgtPos_Get/1 -> Terminator_5/1
  VIPR557TrgtPos_Get/2 -> Terminator_6/1
  VIPR557TrgtPos_Get/4 -> Terminator_7/1
  VIPR557TrgtPos_Get/5 -> Terminator_8/1
  VIPRExit557TrgtPos_Get/1 -> Terminator_9/1
  VIPRExit557TrgtPos_Get/2 -> Terminator_10/1
  VIPRExit557TrgtPos_Get/4 -> Terminator_11/1
  VIPRExit557TrgtPos_Get/5 -> Terminator_12/1
  VIPRExit557TrgtPos_Get/6 -> Terminator_13/1
  VIPRExit557TrgtPos_Get/7 -> Terminator_14/1
  VIPRExit557TrgtPos_Get/8 -> Terminator_15/1
  VIPRExit557TrgtPos_Get/9 -> Terminator_16/1
  VIPRExit557TrgtPos_Get/10 -> Terminator_17/1
  VIPRExit557TrgtPos_Get/11 -> Terminator_18/1
  TrgtPosSelcNo4sMd1/1 -> Md8R2RLgrstUpwdDnwdTrgtPosCalib_TrgtPosArray_write/1
  TrgtPosSelcNo4sMd2/1 -> Md9R2RLgrstUpwdDnwdTrgtPosCalib_TrgtPosArray_write/1
  [Is6s] -> TrgtPosSelcNo4sMd1/1
  [Is6s] -> TrgtPosSelcNo4sMd2/1
  Constant/1 -> TrgtPosSelcNo4sMd1/2
  Constant1/1 -> TrgtPosSelcNo4sMd1/3
  Constant2/1 -> TrgtPosSelcNo4sMd1/4
  PA_KeSMSwAcsMd8SecRwRtStLgrstUpwdPos_Val/1 -> TrgtPosSelcNo4sMd1/5
  PA_KeSMSwAcsMd8SecRwRtStLgrstUpwdPosMax_Val/1 -> TrgtPosSelcNo4sMd1/6
  PA_KeSMSwAcsMd8SecRwRtStLgrstUpwdPosMin_Val/1 -> TrgtPosSelcNo4sMd1/7
  Constant5/1 -> TrgtPosSelcNo4sMd2/4
  Constant4/1 -> TrgtPosSelcNo4sMd2/3
  Constant3/1 -> TrgtPosSelcNo4sMd2/2
  PA_KeSMSwAcsMd9SecRwRtStLgrstUpwdPos_Val/1 -> TrgtPosSelcNo4sMd2/5
  PA_KeSMSwAcsMd9SecRwRtStLgrstUpwdPosMax_Val/1 -> TrgtPosSelcNo4sMd2/6
  PA_KeSMSwAcsMd9SecRwRtStLgrstUpwdPosMin_Val/1 -> TrgtPosSelcNo4sMd2/7

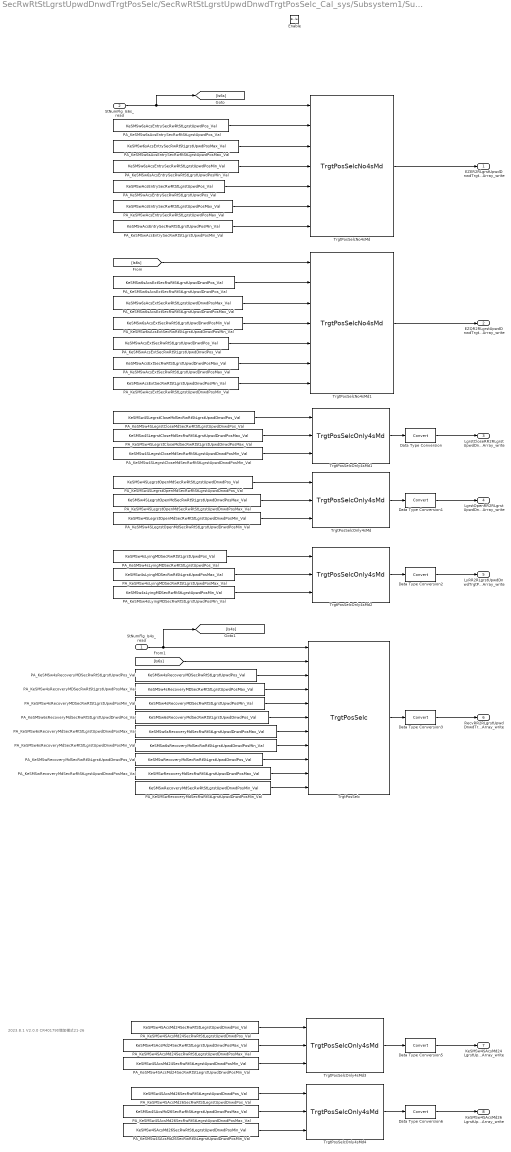
== system SecRwRtStLgrstUpwdDnwdTrgtPosSelc/SecRwRtStLgrstUpwdDnwdTrgtPosSelc_Cal_sys/Subsystem1/Subsystem ==
  note: 2023.8.1 V2.0.0 CR401790 增加模式21-26
  StNumFlg_Is4s_read : Inport
  StNumFlg_Is6s_read : Inport  Port=2
  Enable : EnablePort
  Data Type Conversion{,1..3,5..6} (6 alike) : DataTypeConversion
  PA_KeSMSw4SAcsMd24SecRwRtStLegrstUpwdDnwdPosMax_Val : Constant  Value=KeSMSw4SAcsMd24SecRwRtStLegrstUpwdDnwdPosMax_Val
  PA_KeSMSw4SAcsMd24SecRwRtStLegrstUpwdDnwdPosMin_Val : Constant  Value=KeSMSw4SAcsMd24SecRwRtStLegrstUpwdDnwdPosMin_Val
  PA_KeSMSw4SAcsMd24SecRwRtStLegrstUpwdDnwdPos_Val : Constant  Value=KeSMSw4SAcsMd24SecRwRtStLegrstUpwdDnwdPos_Val
  PA_KeSMSw4SAcsMd26SecRwRtStLegrstUpwdDnwdPosMax_Val : Constant  Value=KeSMSw4SAcsMd26SecRwRtStLegrstUpwdDnwdPosMax_Val
  PA_KeSMSw4SAcsMd26SecRwRtStLegrstUpwdDnwdPosMin_Val : Constant  Value=KeSMSw4SAcsMd26SecRwRtStLegrstUpwdDnwdPosMin_Val
  PA_KeSMSw4SAcsMd26SecRwRtStLegrstUpwdDnwdPos_Val : Constant  Value=KeSMSw4SAcsMd26SecRwRtStLegrstUpwdDnwdPos_Val
  PA_KeSMSw4SLegrstCloseMdSecRwRtStLgrstUpwdDnwdPosMax_Val : Constant  Value=KeSMSw4SLegrstCloseMdSecRwRtStLgrstUpwdDnwdPosMax_Val
  PA_KeSMSw4SLegrstCloseMdSecRwRtStLgrstUpwdDnwdPosMin_Val : Constant  Value=KeSMSw4SLegrstCloseMdSecRwRtStLgrstUpwdDnwdPosMin_Val
  PA_KeSMSw4SLegrstCloseMdSecRwRtStLgrstUpwdDnwdPos_Val : Constant  Value=KeSMSw4SLegrstCloseMdSecRwRtStLgrstUpwdDnwdPos_Val
  PA_KeSMSw4SLegrstOpenMdSecRwRtStLgrstUpwdDnwdPosMax_Val : Constant  Value=KeSMSw4SLegrstOpenMdSecRwRtStLgrstUpwdDnwdPosMax_Val
  PA_KeSMSw4SLegrstOpenMdSecRwRtStLgrstUpwdDnwdPosMin_Val : Constant  Value=KeSMSw4SLegrstOpenMdSecRwRtStLgrstUpwdDnwdPosMin_Val
  PA_KeSMSw4SLegrstOpenMdSecRwRtStLgrstUpwdDnwdPos_Val : Constant  Value=KeSMSw4SLegrstOpenMdSecRwRtStLgrstUpwdDnwdPos_Val
  PA_KeSMSw4sLyingMDSecRwRtStLgrstUpwdPosMax_Val : Constant  Value=KeSMSw4sLyingMDSecRwRtStLgrstUpwdPosMax_Val
  PA_KeSMSw4sLyingMDSecRwRtStLgrstUpwdPosMin_Val : Constant  Value=KeSMSw4sLyingMDSecRwRtStLgrstUpwdPosMin_Val
  PA_KeSMSw4sLyingMDSecRwRtStLgrstUpwdPos_Val : Constant  Value=KeSMSw4sLyingMDSecRwRtStLgrstUpwdPos_Val
  PA_KeSMSw4sRecoveryMDSecRwRtStLgrstUpwdPosMax_Val : Constant  Value=KeSMSw4sRecoveryMDSecRwRtStLgrstUpwdPosMax_Val
  PA_KeSMSw4sRecoveryMDSecRwRtStLgrstUpwdPosMin_Val : Constant  Value=KeSMSw4sRecoveryMDSecRwRtStLgrstUpwdPosMin_Val
  PA_KeSMSw4sRecoveryMDSecRwRtStLgrstUpwdPos_Val : Constant  Value=KeSMSw4sRecoveryMDSecRwRtStLgrstUpwdPos_Val
  PA_KeSMSw6sAcsEntrySecRwRtStLgrstUpwdPosMax_Val : Constant  Value=KeSMSw6sAcsEntrySecRwRtStLgrstUpwdPosMax_Val
  PA_KeSMSw6sAcsEntrySecRwRtStLgrstUpwdPosMin_Val : Constant  Value=KeSMSw6sAcsEntrySecRwRtStLgrstUpwdPosMin_Val
  PA_KeSMSw6sAcsEntrySecRwRtStLgrstUpwdPos_Val : Constant  Value=KeSMSw6sAcsEntrySecRwRtStLgrstUpwdPos_Val
  PA_KeSMSw6sAcsExtSecRwRtStLgrstUpwdDnwdPosMax_Val : Constant  Value=KeSMSw6sAcsExtSecRwRtStLgrstUpwdDnwdPosMax_Val
  PA_KeSMSw6sAcsExtSecRwRtStLgrstUpwdDnwdPosMin_Val : Constant  Value=KeSMSw6sAcsExtSecRwRtStLgrstUpwdDnwdPosMin_Val
  PA_KeSMSw6sAcsExtSecRwRtStLgrstUpwdDnwdPos_Val : Constant  Value=KeSMSw6sAcsExtSecRwRtStLgrstUpwdDnwdPos_Val
  PA_KeSMSw6sRecoveryMdSecRwRtStLgrstUpwdDnwdPosMax_Val : Constant  Value=KeSMSw6sRecoveryMdSecRwRtStLgrstUpwdDnwdPosMax_Val
  PA_KeSMSw6sRecoveryMdSecRwRtStLgrstUpwdDnwdPosMin_Val : Constant  Value=KeSMSw6sRecoveryMdSecRwRtStLgrstUpwdDnwdPosMin_Val
  PA_KeSMSw6sRecoveryMdSecRwRtStLgrstUpwdDnwdPos_Val : Constant  Value=KeSMSw6sRecoveryMdSecRwRtStLgrstUpwdDnwdPos_Val
  PA_KeSMSwAcsEntrySecRwRtStLgrstUpwdPosMax_Val : Constant  Value=KeSMSwAcsEntrySecRwRtStLgrstUpwdPosMax_Val
  PA_KeSMSwAcsEntrySecRwRtStLgrstUpwdPosMin_Val : Constant  Value=KeSMSwAcsEntrySecRwRtStLgrstUpwdPosMin_Val
  PA_KeSMSwAcsEntrySecRwRtStLgrstUpwdPos_Val : Constant  Value=KeSMSwAcsEntrySecRwRtStLgrstUpwdPos_Val
  PA_KeSMSwAcsExtSecRwRtStLgrstUpwdDnwdPosMax_Val : Constant  Value=KeSMSwAcsExtSecRwRtStLgrstUpwdDnwdPosMax_Val
  PA_KeSMSwAcsExtSecRwRtStLgrstUpwdDnwdPosMin_Val : Constant  Value=KeSMSwAcsExtSecRwRtStLgrstUpwdDnwdPosMin_Val
  PA_KeSMSwAcsExtSecRwRtStLgrstUpwdDnwdPos_Val : Constant  Value=KeSMSwAcsExtSecRwRtStLgrstUpwdDnwdPos_Val
  PA_KeSMSwRecoveryMdSecRwRtStLgrstUpwdDnwdPosMax_Val : Constant  Value=KeSMSwRecoveryMdSecRwRtStLgrstUpwdDnwdPosMax_Val
  PA_KeSMSwRecoveryMdSecRwRtStLgrstUpwdDnwdPosMin_Val : Constant  Value=KeSMSwRecoveryMdSecRwRtStLgrstUpwdDnwdPosMin_Val
  PA_KeSMSwRecoveryMdSecRwRtStLgrstUpwdDnwdPos_Val : Constant  Value=KeSMSwRecoveryMdSecRwRtStLgrstUpwdDnwdPos_Val
  TrgtPosSelc : TrgtPosSelcLib/TrgtPosSelc  SystemSampleTime=-1
  TrgtPosSelcNo4sMd : TrgtPosSelcLib/TrgtPosSelcNo4sMd  SystemSampleTime=-1
  TrgtPosSelcNo4sMd1 : TrgtPosSelcLib/TrgtPosSelcNo4sMd  SystemSampleTime=-1
  TrgtPosSelcOnly4sMd{,1..4} (5 alike) : TrgtPosSelcLib/TrgtPosSelcOnly4sMd  SystemSampleTime=-1
  EZER2RLgrstUpwdDnwdTrgtPosCalib_TrgtPosArray_write : Outport
      settings: EnsureOutportIsVirtual=on
  EZQR2RLgrstUpwdDnwdTrgtPosCalib_TrgtPosArray_write : Outport  Port=2
      settings: EnsureOutportIsVirtual=on
  LgrstCloseRR2RLgrstUpwdDnwdTrgtPosCalib_TrgtPosArray_write : Outport  Port=3
  LgrstOpenRR2RLgrstUpwdDnwdTrgtPosCalib_TrgtPosArray_write : Outport  Port=4
  LyRR2RLgrstUpwdDnwdTrgtPosCalib_TrgtPosArray_write : Outport  Port=5
  RecvRR2RLgrstUpwdDnwdTrgtPosCalib_TrgtPosArray_write : Outport  Port=6
  KeSMSw4SAcsMd24LgrstUpwdDnwdTrgtPosCalib_TrgtPosArray_write : Outport  Port=7
  KeSMSw4SAcsMd26LgrstUpwdDnwdTrgtPosCalib_TrgtPosArray_write : Outport  Port=8
  wires:
  PA_KeSMSw6sRecoveryMdSecRwRtStLgrstUpwdDnwdPos_Val/1 -> TrgtPosSelc/6
  PA_KeSMSwAcsEntrySecRwRtStLgrstUpwdPosMax_Val/1 -> TrgtPosSelcNo4sMd/6
  TrgtPosSelcNo4sMd/1 -> EZER2RLgrstUpwdDnwdTrgtPosCalib_TrgtPosArray_write/1
  PA_KeSMSw6sRecoveryMdSecRwRtStLgrstUpwdDnwdPosMin_Val/1 -> TrgtPosSelc/8
  PA_KeSMSw4sRecoveryMDSecRwRtStLgrstUpwdPosMin_Val/1 -> TrgtPosSelc/5
  PA_KeSMSwRecoveryMdSecRwRtStLgrstUpwdDnwdPos_Val/1 -> TrgtPosSelc/9
  TrgtPosSelcOnly4sMd2/1 -> Data Type Conversion2/1
  PA_KeSMSw4SLegrstOpenMdSecRwRtStLgrstUpwdDnwdPosMax_Val/1 -> TrgtPosSelcOnly4sMd/2
  PA_KeSMSwAcsEntrySecRwRtStLgrstUpwdPos_Val/1 -> TrgtPosSelcNo4sMd/5
  PA_KeSMSwAcsEntrySecRwRtStLgrstUpwdPosMin_Val/1 -> TrgtPosSelcNo4sMd/7
  PA_KeSMSw4SLegrstOpenMdSecRwRtStLgrstUpwdDnwdPosMin_Val/1 -> TrgtPosSelcOnly4sMd/3
  PA_KeSMSw6sAcsEntrySecRwRtStLgrstUpwdPos_Val/1 -> TrgtPosSelcNo4sMd/2
  PA_KeSMSw6sAcsEntrySecRwRtStLgrstUpwdPosMax_Val/1 -> TrgtPosSelcNo4sMd/3
  TrgtPosSelcOnly4sMd1/1 -> Data Type Conversion/1
  PA_KeSMSwRecoveryMdSecRwRtStLgrstUpwdDnwdPosMax_Val/1 -> TrgtPosSelc/10
  StNumFlg_Is4s_read/1 -> [Is4s], TrgtPosSelc/1
  PA_KeSMSw4SLegrstOpenMdSecRwRtStLgrstUpwdDnwdPos_Val/1 -> TrgtPosSelcOnly4sMd/1
  PA_KeSMSw6sRecoveryMdSecRwRtStLgrstUpwdDnwdPosMax_Val/1 -> TrgtPosSelc/7
  StNumFlg_Is6s_read/1 -> [Is6s], TrgtPosSelcNo4sMd/1
  PA_KeSMSw6sAcsEntrySecRwRtStLgrstUpwdPosMin_Val/1 -> TrgtPosSelcNo4sMd/4
  PA_KeSMSw4sRecoveryMDSecRwRtStLgrstUpwdPos_Val/1 -> TrgtPosSelc/3
  PA_KeSMSwRecoveryMdSecRwRtStLgrstUpwdDnwdPosMin_Val/1 -> TrgtPosSelc/11
  [Is6s] -> TrgtPosSelc/2
  PA_KeSMSw4sRecoveryMDSecRwRtStLgrstUpwdPosMax_Val/1 -> TrgtPosSelc/4
  TrgtPosSelcNo4sMd1/1 -> EZQR2RLgrstUpwdDnwdTrgtPosCalib_TrgtPosArray_write/1
  TrgtPosSelcOnly4sMd/1 -> Data Type Conversion1/1
  TrgtPosSelc/1 -> Data Type Conversion3/1
  [Is6s] -> TrgtPosSelcNo4sMd1/1
  PA_KeSMSw4SLegrstCloseMdSecRwRtStLgrstUpwdDnwdPosMin_Val/1 -> TrgtPosSelcOnly4sMd1/3
  PA_KeSMSw4SLegrstCloseMdSecRwRtStLgrstUpwdDnwdPosMax_Val/1 -> TrgtPosSelcOnly4sMd1/2
  PA_KeSMSw4SLegrstCloseMdSecRwRtStLgrstUpwdDnwdPos_Val/1 -> TrgtPosSelcOnly4sMd1/1
  PA_KeSMSw4sLyingMDSecRwRtStLgrstUpwdPosMin_Val/1 -> TrgtPosSelcOnly4sMd2/3
  PA_KeSMSw4sLyingMDSecRwRtStLgrstUpwdPosMax_Val/1 -> TrgtPosSelcOnly4sMd2/2
  PA_KeSMSw4sLyingMDSecRwRtStLgrstUpwdPos_Val/1 -> TrgtPosSelcOnly4sMd2/1
  PA_KeSMSw6sAcsExtSecRwRtStLgrstUpwdDnwdPosMax_Val/1 -> TrgtPosSelcNo4sMd1/3
  PA_KeSMSw6sAcsExtSecRwRtStLgrstUpwdDnwdPos_Val/1 -> TrgtPosSelcNo4sMd1/2
  PA_KeSMSw6sAcsExtSecRwRtStLgrstUpwdDnwdPosMin_Val/1 -> TrgtPosSelcNo4sMd1/4
  PA_KeSMSwAcsExtSecRwRtStLgrstUpwdDnwdPosMax_Val/1 -> TrgtPosSelcNo4sMd1/6
  PA_KeSMSwAcsExtSecRwRtStLgrstUpwdDnwdPos_Val/1 -> TrgtPosSelcNo4sMd1/5
  PA_KeSMSwAcsExtSecRwRtStLgrstUpwdDnwdPosMin_Val/1 -> TrgtPosSelcNo4sMd1/7
  Data Type Conversion/1 -> LgrstCloseRR2RLgrstUpwdDnwdTrgtPosCalib_TrgtPosArray_write/1
  Data Type Conversion1/1 -> LgrstOpenRR2RLgrstUpwdDnwdTrgtPosCalib_TrgtPosArray_write/1
  Data Type Conversion2/1 -> LyRR2RLgrstUpwdDnwdTrgtPosCalib_TrgtPosArray_write/1
  PA_KeSMSw4SAcsMd24SecRwRtStLegrstUpwdDnwdPos_Val/1 -> TrgtPosSelcOnly4sMd3/1
  PA_KeSMSw4SAcsMd26SecRwRtStLegrstUpwdDnwdPos_Val/1 -> TrgtPosSelcOnly4sMd4/1
  TrgtPosSelcOnly4sMd3/1 -> Data Type Conversion5/1
  TrgtPosSelcOnly4sMd4/1 -> Data Type Conversion6/1
  PA_KeSMSw4SAcsMd26SecRwRtStLegrstUpwdDnwdPosMax_Val/1 -> TrgtPosSelcOnly4sMd4/2
  PA_KeSMSw4SAcsMd26SecRwRtStLegrstUpwdDnwdPosMin_Val/1 -> TrgtPosSelcOnly4sMd4/3
  PA_KeSMSw4SAcsMd24SecRwRtStLegrstUpwdDnwdPosMax_Val/1 -> TrgtPosSelcOnly4sMd3/2
  PA_KeSMSw4SAcsMd24SecRwRtStLegrstUpwdDnwdPosMin_Val/1 -> TrgtPosSelcOnly4sMd3/3
  Data Type Conversion3/1 -> RecvRR2RLgrstUpwdDnwdTrgtPosCalib_TrgtPosArray_write/1
  Data Type Conversion5/1 -> KeSMSw4SAcsMd24LgrstUpwdDnwdTrgtPosCalib_TrgtPosArray_write/1
  Data Type Conversion6/1 -> KeSMSw4SAcsMd26LgrstUpwdDnwdTrgtPosCalib_TrgtPosArray_write/1
